simulink model "chap11_2sim"  (Simulink 7.0)
settings: Solver=ode45  StartTime=0.0  StopTime=50  RelTol=1e-3
settings Model: Creator=eleliuj  LastModifiedBy=eleliuj
settings DataIOCC: SignalLoggingName=sigsOut
settings DebuggingCC: SaveWithParameterizedLinksMsg=none  SignalResolutionControl=TryResolveAllWithWarning  SolverPrmCheckMsg=none  MultiTaskDSMMsg=warning  MultiTaskCondExecSysMsg=none  StrictBusMsg=None
settings HardwareCC: TargetUnknown=on
settings RTWCC: IncludeERTFirstTime=on

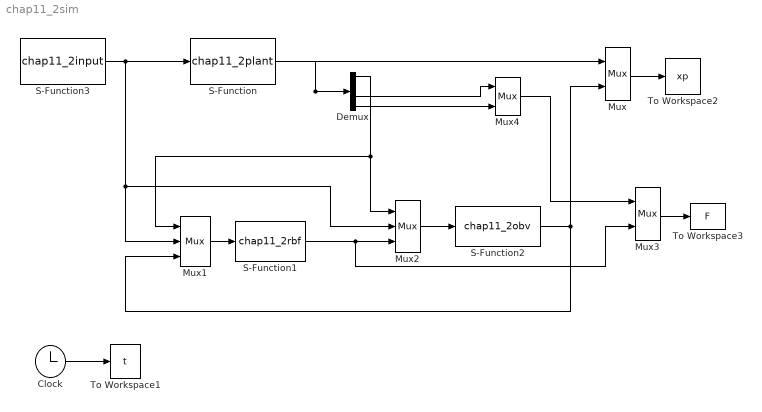
== system chap11_2sim ==
  Clock : Clock
      settings: Decimation=10
  Demux : Demux
  Mux : Mux  Inputs=2
  Mux1 : Mux  Inputs=3
  Mux2 : Mux  Inputs=3
  Mux3 : Mux  Inputs=2
  Mux4 : Mux  Inputs=2
  S-Function : S-Function  FunctionName=chap11_2plant
  S-Function1 : S-Function  FunctionName=chap11_2rbf
  S-Function2 : S-Function  FunctionName=chap11_2obv
  S-Function3 : S-Function  FunctionName=chap11_2input
  To Workspace1 : ToWorkspace  VariableName=t  SampleTime=-1  SaveFormat=Array
  To Workspace2 : ToWorkspace  VariableName=xp  SampleTime=-1  SaveFormat=Array
  To Workspace3 : ToWorkspace  VariableName=F  SampleTime=-1  SaveFormat=Array
  wires:
  S-Function3/1 -> S-Function/1, Mux2/2, Mux1/2
  Clock/1 -> To Workspace1/1
  Mux/1 -> To Workspace2/1
  S-Function2/1 -> Mux/2, Mux1/3
  Mux1/1 -> S-Function1/1
  Mux2/1 -> S-Function2/1
  S-Function1/1 -> Mux2/3, Mux3/2
  S-Function/1 -> Mux/1, Demux/1
  Demux/1 -> Mux2/1, Mux1/1
  Mux3/1 -> To Workspace3/1
  Mux4/1 -> Mux3/1
  Demux/3 -> Mux4/1
  Demux/4 -> Mux4/2
